simulink model "controller_attitude"  (R2020a)
settings: Solver=FixedStepAuto  StartTime=0.0  StopTime=10.0  FixedStep=1/sim_freq  RelTol=1e-3
undefined symbols (not defined in the file): sim_freq
libraries: sharedtransform x2
settings Model: Creator=francois  LastModifiedBy=murray

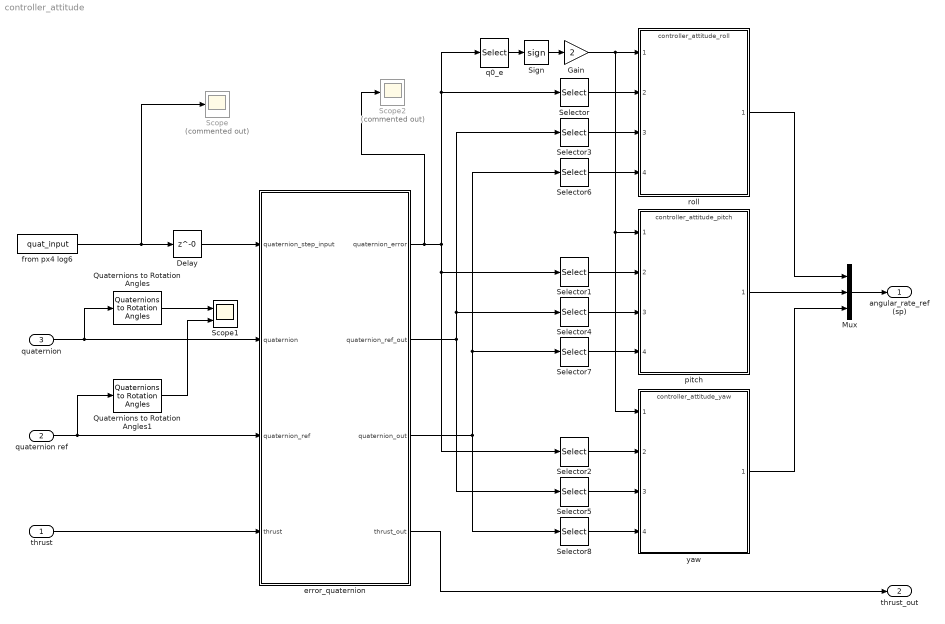
== system controller_attitude ==
  "thrust " : Inport  SampleTime=1/sim_freq
  quaternion ref : Inport  Port=2  SampleTime=1/sim_freq
  "quaternion " : Inport  Port=3  SampleTime=1/sim_freq
  Delay : Delay  DelayLength=0
  Gain : Gain  Gain=2
  Mux : Mux  Inputs=3
  Quaternions to Rotation Angles : sharedtransform/Quaternions to Rotation Angles  rotationOrder=ZYX  aMode=aMode
      settings: SourceProductBaseCode=AE,PW,MT,VE,VP
  Quaternions to Rotation Angles1 : sharedtransform/Quaternions to Rotation Angles  rotationOrder=ZYX  aMode=aMode
      settings: SourceProductBaseCode=AE,PW,MT,VE,VP
  Scope : Scope  Commented=on
  Scope1 : Scope  NumInputPorts=2
  Scope2 : Scope  Commented=on
  Selector : Selector  InputPortWidth=4  IndexOptions=Index vector (dialog)  Indices=2  OutputSizes=1
  Selector1 : Selector  InputPortWidth=4  IndexOptions=Index vector (dialog)  Indices=3  OutputSizes=1
  Selector2 : Selector  InputPortWidth=4  IndexOptions=Index vector (dialog)  Indices=4  OutputSizes=1
  Selector3 : Selector  InputPortWidth=4  IndexOptions=Index vector (dialog)  Indices=2  OutputSizes=1
  Selector4 : Selector  InputPortWidth=4  IndexOptions=Index vector (dialog)  Indices=3  OutputSizes=1
  Selector5 : Selector  InputPortWidth=4  IndexOptions=Index vector (dialog)  Indices=4  OutputSizes=1
  Selector6 : Selector  InputPortWidth=4  IndexOptions=Index vector (dialog)  Indices=2  OutputSizes=1
  Selector7 : Selector  InputPortWidth=4  IndexOptions=Index vector (dialog)  Indices=3  OutputSizes=1
  Selector8 : Selector  InputPortWidth=4  IndexOptions=Index vector (dialog)  Indices=4  OutputSizes=1
  Sign : Signum
  "error_quaternion " : MATLAB Function  TreatAsAtomicUnit=on  SystemSampleTime=1/sim_freq
  from px4 log6 : FromWorkspace  VariableName=quat_input
  pitch : ModelReference  ModelNameDialog=controller_attitude_pitch.slx  SimulationMode=Normal  ModelReferenceVersion=1.15
  q0_e : Selector  InputPortWidth=4  IndexOptions=Index vector (dialog)  Indices=1  OutputSizes=1
  roll : ModelReference  ModelNameDialog=controller_attitude_roll.slx  SimulationMode=Normal  ModelReferenceVersion=1.11
  yaw : ModelReference  ModelNameDialog=controller_attitude_yaw.slx  SimulationMode=Normal  ModelReferenceVersion=1.13
  angular_rate_ref (sp) : Outport
  thrust_out : Outport  Port=2
  wires:
  roll/1 -> Mux/1
  pitch/1 -> Mux/2
  yaw/1 -> Mux/3
  Mux/1 -> angular_rate_ref (sp)/1
  from px4 log6/1 -> Scope/1, Delay/1
  Delay/1 -> "error_quaternion "/1(quaternion_step_input)
  "quaternion "/1 -> Quaternions to Rotation Angles/1, "error_quaternion "/2(quaternion)
  quaternion ref/1 -> Quaternions to Rotation Angles1/1, "error_quaternion "/3(quaternion_ref)
  "thrust "/1 -> "error_quaternion "/4(thrust)
  Quaternions to Rotation Angles/1 -> Scope1/1
  Quaternions to Rotation Angles1/1 -> Scope1/2
  "error_quaternion "/1(quaternion_error) -> Scope2/1, Selector/1, q0_e/1, Selector1/1, Selector2/1
  q0_e/1 -> Sign/1
  Sign/1 -> Gain/1
  Gain/1 -> yaw/1, pitch/1, roll/1
  Selector/1 -> roll/2
  Selector1/1 -> pitch/2
  Selector2/1 -> yaw/2
  "error_quaternion "/2(quaternion_ref_out) -> Selector4/1, Selector3/1, Selector5/1
  Selector4/1 -> pitch/3
  Selector3/1 -> roll/3
  Selector5/1 -> yaw/3
  Selector6/1 -> roll/4
  Selector7/1 -> pitch/4
  Selector8/1 -> yaw/4
  "error_quaternion "/3(quaternion_out) -> Selector8/1, Selector7/1, Selector6/1
  "error_quaternion "/4(thrust_out) -> thrust_out/1

== matlab function controller_attitude/error_quaternion  ==
  data: quaternion_step_input input; quaternion_error output size=[1 4]; quaternion input; quaternion_ref input; thrust input; quaternion_ref_out output; quaternion_out output; thrust_out output; hover_perc parameter
function [quaternion_error, quaternion_ref_out, quaternion_out, thrust_out] = error_quat(quaternion_step_input, quaternion, quaternion_ref, thrust, hover_perc)
    if quaternion_step_input ~= [0; 0; 0; 0]
        quaternion_error = quatmultiply([quaternion(1) -quaternion(2) -quaternion(3) -quaternion(4)]./norm(quaternion), quaternion_step_input');
        quaternion_ref_out = quaternion_step_input; 
        quaternion_out = sign(quaternion_step_input(1)) .* quaternion;
        
        thrust_out = hover_perc;
    else
        if quaternion_ref == [0; 0; 0; 0]
           quaternion_ref = [1; 0; 0; 0];
        end
        quaternion_error = quatmultiply([quaternion(1) -quaternion(2) -quaternion(3) -quaternion(4)]./norm(quaternion), quaternion_ref');
        quaternion_ref_out = quaternion_ref; 
        quaternion_out = sign(quaternion_ref(1)) .* quaternion;
    
        thrust_out = thrust;
    end
end
